simulink model "noise2"  (R2021a)
settings: Solver=VariableStepAuto  StartTime=0.0  StopTime=2  RelTol=1e-3
libraries: dspxfrm3 x2, commchan3 x1, dsparch4 x1
settings Model: Creator=Safir  LastModifiedBy=Safir

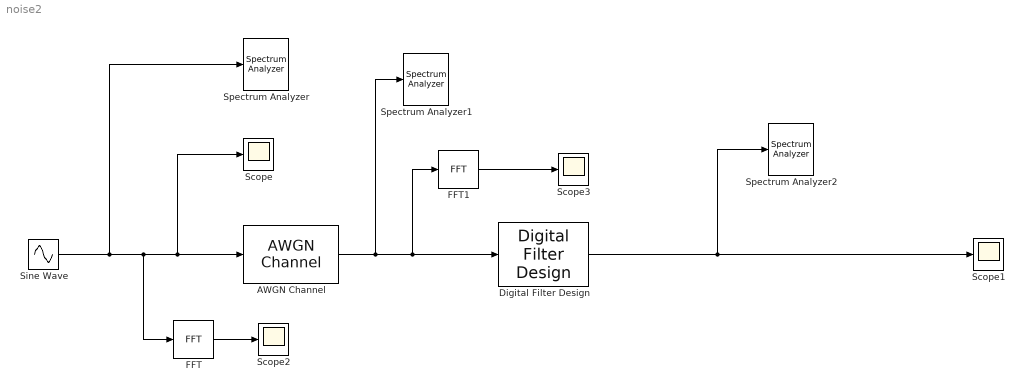
== system noise2 ==
  AWGN Channel : commchan3/AWGN Channel  InputProcessing=Columns as channels (frame based)  seed=67  noiseMode="Signal to noise ratio  (SNR)"  EbNodB=10  EsNodB=10  SNRdB=1  bitsPerSym=1  Ps=1  Tsym=1  variance=1
  Digital Filter Design : dsparch4/Digital Filter Design  mwdsp_browser_bugfix_var=off
  FFT : dspxfrm3/FFT  FFTImplementation=Auto  CompMethod=Table lookup  TableOpt=NEW  TableOptActive=Speed  BitRevOrder=off  Normalize=off  InheritFFTLength=on  FFTLength=64  WrapInput=on  roundingMode=Floor  overflowMode=off  firstCoeffDataTypeStr=Inherit: Same word length as input  firstCoeffLastDataTypeStr=Inherit: Same word length as input  outputMin=[]  outputMax=[]
  FFT1 : dspxfrm3/FFT  FFTImplementation=Auto  CompMethod=Table lookup  TableOpt=NEW  TableOptActive=Speed  BitRevOrder=off  Normalize=off  InheritFFTLength=on  FFTLength=64  WrapInput=on  roundingMode=Floor  overflowMode=off  firstCoeffDataTypeStr=Inherit: Same word length as input  firstCoeffLastDataTypeStr=Inherit: Same word length as input  outputMin=[]  outputMax=[]
  Scope{,1..3} (4 alike) : Scope
  Sine Wave : Sin  Frequency=2*pi*1000  SampleTime=1.25e-4
  Spectrum Analyzer : SpectrumAnalyzer
  Spectrum Analyzer1 : SpectrumAnalyzer
  Spectrum Analyzer2 : SpectrumAnalyzer
  wires:
  Sine Wave/1 -> Spectrum Analyzer/1, FFT/1, Scope/1, AWGN Channel/1
  AWGN Channel/1 -> Spectrum Analyzer1/1, FFT1/1, Digital Filter Design/1
  Digital Filter Design/1 -> Spectrum Analyzer2/1, Scope1/1
  FFT/1 -> Scope2/1
  FFT1/1 -> Scope3/1
